simulink subsystem "EPOS4"  (R2021b)
settings: Solver=VariableStepAuto  StartTime=0.0  StopTime=10.0  RelTol=1e-3
undefined symbols (not defined in the file): DiscIntNeverNeededParam, Ts_Vel, x3001_5, x30A0_1, x30A0_2, x30A2_1, x30A2_2, x30A3_1, x30A3_2, x30A3_3, x30A3_4, x30A3_5, x520886_ICont, x607325_RotIner, x607325_RotOmgMax, x607325_Torq, x607325_TorqConst, x607325_VNom
libraries: fl_lib x4, nesl_utility x3, ee_lib x2, slpidlib x1
settings Model: Creator=khoi  LastModifiedBy=khoi
settings SolverCC: AlgebraicLoopSolver=TrustRegion
settings DebuggingCC: SFMachineParentedDataDiag=warning

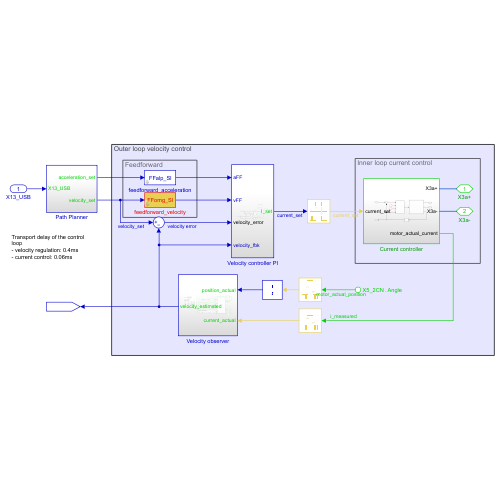
[thumbnail: Simulink's stored preview of the top-level diagram]
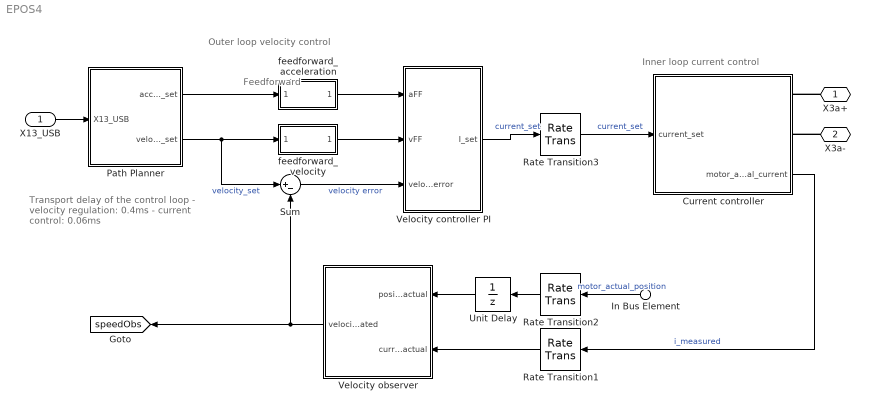
== system EPOS4 ==
  note: Outer loop velocity control
  note: Feedforward
  note: Inner loop current control
  note: Transport delay of the control loop
      | - velocity regulation: 0.4ms
      | - current control: 0.06ms
  X13_USB : Inport  OutDataTypeStr=double
  In Bus Element : Inport  Port=2  PortName=X5_2CN  Element=Angle
  Current controller : Subsystem
      settings: PortSchema="{\"entries\":[{\"content\":{\"sides\":[{\"content\":{\"connectorIds\":[\"In1\"]},\"type\":\"ConnectorPlacement.EquallySpacedRectSide\",\"uuid\":\"3e5704e1-1bc4-4e0c-b161-9fade073eb22\"},{\"content\":{\"connectorIds\":[\"RConn1\",\"RConn2\",\"Out1\"],\"side\":\"RIGHT\"},\"type\":\"ConnectorPlacement.EquallySpacedRectSide\",\"uuid\":\"52ff2dfd-ee16-417d-b7e8-bdd096001b9c\"},{\"content\":{\"connectorIds\":[],\"side\":\"TOP\"},\"type\":\"ConnectorPlacement.EquallySpacedRectSide\",\"uuid\":\"337a9011-df50-4122-8385-03af17ddf6d7\"}]},\"type\":\"ConnectorPlacement.EquallySpacedConnector\",\"uuid\":\"8d932baa-b47a-45b5-987d-77891fcdc649\"}],\"packageUris\":[\"http://schema.mathworks.com/mf0/Connector/R2020b\"],\"version\":\"1.0\"}"
  Path Planner : Subsystem
  Rate Transition1 : RateTransition  Deterministic=off  OutPortSampleTime=Ts_Vel
  Rate Transition2 : RateTransition  Deterministic=off  OutPortSampleTime=Ts_Vel
  Rate Transition3 : RateTransition  Deterministic=off  OutPortSampleTime=Ts_Curr
  Sum : Sum  Inputs=|+-
  Unit Delay : UnitDelay  SampleTime=Ts_Vel  HasFrameUpgradeWarning=on
  Velocity controller PI : Subsystem
  Velocity observer : Subsystem
  feedforward_acceleration : Subsystem  mask{Value=80}
      mask prompts: Value "Load inertia (g*cm^2)"
      mask TypeOptions Value: Constant1/Value
      mask DialogControl DescGroupVar Prompt: Feedforward acceleration
      mask Display: disp('FFalp_SI')
  feedforward_velocity : Subsystem  mask{Value=0}
      mask prompts: Value "Total friction proportional factor"
      mask DialogControl DescGroupVar Prompt: Feedforward velocity
      mask Display: disp('FFomg_SI')
  X3a+ : PMIOPort  Side=Left
  X3a- : PMIOPort  Port=2  Side=Left
  tag scope: speedObs=global
  wires:
  Path Planner/2(velocity_set) -> feedforward_velocity/1(X13_USB), Sum/1  "velocity_set"
  Path Planner/1(acceleration_set) -> feedforward_acceleration/1(X13_USB)
  feedforward_acceleration/1(Out1) -> Velocity controller PI/1(aFF)
  In Bus Element/1 -> Rate Transition2/1  "motor_actual_position"
  Current controller/1(motor_actual_current) -> Rate Transition1/1  "i_measured"
  feedforward_velocity/1(Out1) -> Velocity controller PI/2(vFF)
  Velocity controller PI/1(I_set) -> Rate Transition3/1  "current_set"
  Rate Transition3/1 -> Current controller/1(current_set)  "current_set"
  X13_USB/1 -> Path Planner/1(X13_USB)
  Unit Delay/1 -> Velocity observer/1(position_actual)
  Rate Transition2/1 -> Unit Delay/1
  Rate Transition1/1 -> Velocity observer/2(current_actual)
  Velocity observer/1(velocity_estimated) -> Sum/2, [speedObs]
  Sum/1 -> Velocity controller PI/3(velocity_error)  "velocity error"
  connections:
  X3a+/RConn1 -- Current controller/RConn1
  X3a-/RConn1 -- Current controller/RConn2

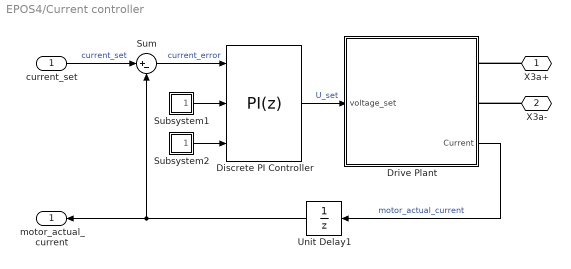
== system EPOS4/Current controller ==
  current_set : Inport  Unit=A
  Discrete PI Controller : slpidlib/PID Controller  Controller=PI  Form=Parallel  TimeDomain=Discrete-time  UseExternalTs=off  SampleTime=-1  IntegratorMethod=Forward Euler  FilterMethod=Forward Euler  ControllerParametersSource=external  P=1  I=1  D=0  UseFilter=on  N=100  TunerSelectOption=Transfer Function Based (PID Tuner App)  InitialConditionSource=internal  InitialConditionForIntegrator=0  InitialConditionForFilter=0  DifferentiatorICPrevScaledInput=0  ExternalReset=none  TrackingMode=off  Kt=0  LimitOutput=on  SatLimitsSource=internal  UpperSaturationLimit=x607325_VNom  LowerSaturationLimit=-x607325_VNom  LinearizeAsGain=off  AntiWindupMode=clamping  Kb=500  POutMin=[]  POutMax=[]  IOutMin=[]  IOutMax=[]  DOutMin=[]  DOutMax=[]  NOutMin=[]  NOutMax=[]  SumOutMin=[]  SumOutMax=[]  SaturationOutMin=[]  SaturationOutMax=[]  PParamMin=[]  PParamMax=[]  IParamMin=[]  IParamMax=[]  DParamMin=[]  DParamMax=[]  NParamMin=[]  NParamMax=[]  KbParamMin=[]  KbParamMax=[]  KtParamMin=[]  KtParamMax=[]  KbOutMin=[]  KbOutMax=[]  KtOutMin=[]  KtOutMax=[]  IntegratorOutMin=[]  IntegratorOutMax=[]  FilterOutMin=[]  FilterOutMax=[]  SumI1OutMin=[]  SumI1OutMax=[]  SumI2OutMin=[]  SumI2OutMax=[]  SumI3OutMin=[]  SumI3OutMax=[]  SumI4OutMin=[]  SumI4OutMax=[]  SumDOutMin=[]  SumDOutMax=[]  DifferentiatorOutMin=[]  DifferentiatorOutMax=[]  FilterDiffOutCoefMin=[]  FilterDiffOutCoefMax=[]  ReciprocalOutMin=[]  ReciprocalOutMax=[]  SumDenOutMin=[]  SumDenOutMax=[]  SumNumOutMin=[]  SumNumOutMax=[]  DivideOutMin=[]  DivideOutMax=[]  UdiffTsProdOutMin=[]  UdiffTsProdOutMax=[]  NTsProdOutMin=[]  NTsProdOutMax=[]  UintegralTsProdOutMin=[]  UintegralTsProdOutMax=[]  UngainTsProdOutMin=[]  UngainTsProdOutMax=[]  IntegratorContinuousStateAttributes=''  IntegratorStateMustResolveToSignalObject=off  IntegratorRTWStateStorageClass=Auto  FilterContinuousStateAttributes=''  FilterStateMustResolveToSignalObject=off  FilterRTWStateStorageClass=Auto  ParallelPVariant=ExternalParameters  IdealPVariant=Disabled  IVariant=ExternalParameters  DVariant=Disabled  IntegratorVariant=Discrete  SatVariant=Enabled  AWVariant=DiscClampingParallel  PCopyVariant=Disabled  TRVariant=Disabled  FdbkBlocksVariant=Forward  IdealPFdbkVariant=Disabled  SatFdbkVariant=Disabled  DerivativeFilterVariant=Disabled  NVariant=Disabled  NCopyVariant=Disabled_SignalSpec  FilterICVariant=Disabled  IntegratorICVariant=InternalICs  ExternalResetVariant=Disabled  TRSumVariant=Passthrough  SumFdbkVariant=Disabled  SumVariant=Sum_PI  TsampFilterVariant=InternalTs  TsampNgainVariant=Passthrough  TsampIntegralVariant=Passthrough  ExternalSaturationOutDataTypeStr=Inherit: Same as second input
  Drive Plant : Subsystem
      settings: PortSchema="{\"entries\":[{\"content\":{\"sides\":[{\"content\":{\"connectorIds\":[\"In1\"]},\"type\":\"ConnectorPlacement.EquallySpacedRectSide\",\"uuid\":\"2af1de9d-8962-474e-8952-77c9402ebadb\"},{\"content\":{\"connectorIds\":[\"RConn1\",\"RConn2\",\"Out1\"],\"side\":\"RIGHT\"},\"type\":\"ConnectorPlacement.EquallySpacedRectSide\",\"uuid\":\"e1a8f025-59c3-4187-9e1a-5d7de5437d6b\"},{\"content\":{\"connectorIds\":[],\"side\":\"TOP\"},\"type\":\"ConnectorPlacement.EquallySpacedRectSide\",\"uuid\":\"98ea0e18-1fc3-4a14-86ec-43c827e86c22\"}]},\"type\":\"ConnectorPlacement.EquallySpacedConnector\",\"uuid\":\"e2751f7d-b1df-4c60-a3ed-7b97aa6d6783\"}],\"packageUris\":[\"http://schema.mathworks.com/mf0/Connector/R2020b\"],\"version\":\"1.0\"}"
      mask Display: disp('Power\ndevice')
  Subsystem1 : Subsystem
  Subsystem2 : Subsystem
  Sum : Sum  Inputs=|+-
  Unit Delay1 : UnitDelay  SampleTime=0.06e-3  HasFrameUpgradeWarning=on
  X3a+ : PMIOPort  Side=Right
  X3a- : PMIOPort  Port=2  Side=Right
  motor_actual_current : Outport  Unit=A
  wires:
  current_set/1 -> Sum/1  "current_set"
  Subsystem2/1(Out1) -> Discrete PI Controller/3
  Subsystem1/1(Out1) -> Discrete PI Controller/2
  Unit Delay1/1 -> Sum/2, motor_actual_current/1
  Sum/1 -> Discrete PI Controller/1  "current_error"
  Discrete PI Controller/1 -> Drive Plant/1(voltage_set)  "U_set"
  Drive Plant/1(Current) -> Unit Delay1/1  "motor_actual_current"
  connections:
  X3a-/RConn1 -- Drive Plant/RConn2
  X3a+/RConn1 -- Drive Plant/RConn1

== system EPOS4/Path Planner ==
  X13_USB : Inport
  Demux : Demux  Outputs=3
  Terminator : Terminator
  acceleration_set : Outport  Unit=rad/s^2
  velocity_set : Outport  Port=2  Unit=rad/s
  wires:
  Demux/2 -> velocity_set/1
  X13_USB/1 -> Demux/1
  Demux/3 -> acceleration_set/1
  Demux/1 -> Terminator/1

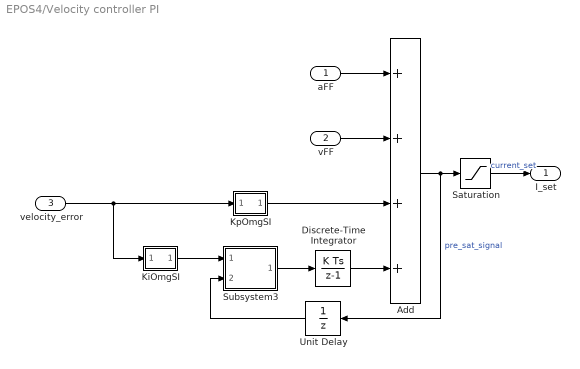
== system EPOS4/Velocity controller PI ==
  aFF : Inport
  vFF : Inport  Port=2
  velocity_error : Inport  Port=3  Unit=rad/s
  Add : Sum  Inputs=++++
  Discrete-Time Integrator : DiscreteIntegrator  SampleTime=-1  ICPrevOutput=DiscIntNeverNeededParam  ICPrevScaledInput=DiscIntNeverNeededParam
  KiOmgSI : Subsystem
  KpOmgSI : Subsystem
  Saturation : Saturate  UpperLimit=x520886_ICont  LowerLimit=-x520886_ICont
  Subsystem3 : Subsystem  mask{UpperValue=x520886_ICont, LowerValue=-x520886_ICont}
      mask prompts: UpperValue "Upper limit"; LowerValue "Lower limit"
      mask TypeOptions UpperValue: Dead Zone/UpperValue
      mask TypeOptions LowerValue: Dead Zone/LowerValue
      mask DialogControl DescGroupVar Prompt: Limit
      mask Display: disp('Anti-\nwindup')
  Unit Delay : UnitDelay  SampleTime=-1  HasFrameUpgradeWarning=on
  I_set : Outport  Unit=A
  wires:
  velocity_error/1 -> KpOmgSI/1(velocity_error), KiOmgSI/1(velocity_set)
  Add/1 -> Saturation/1, Unit Delay/1  "pre_sat_signal"
  KpOmgSI/1(Out1) -> Add/3
  vFF/1 -> Add/2
  KiOmgSI/1(Out1) -> Subsystem3/1(PreInt)
  aFF/1 -> Add/1
  Subsystem3/1(Out1) -> Discrete-Time Integrator/1
  Discrete-Time Integrator/1 -> Add/4
  Unit Delay/1 -> Subsystem3/2(PreSat)
  Saturation/1 -> I_set/1  "current_set"

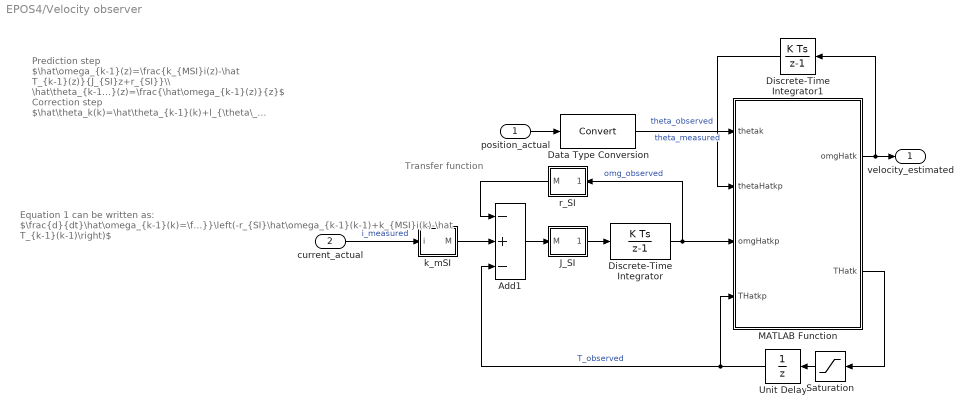
== system EPOS4/Velocity observer ==
  note: Prediction step
      | $\hat\omega_{k-1}(z)=\frac{k_{MSI}i(z)-\hat T_{k-1}(z)}{J_{SI}z+r_{SI}}\\ \hat\theta_{k-1}(z)=\frac{\hat\omega_{k-1}(z)}{z}$
      | Correction step
      | $\hat\theta_k(k)=\hat\theta_{k-1}(k)+l_{\theta\_ SI}\left[\theta(k)-\hat\theta_{k-1}(k)\right]\\ \hat\omega_k(k)=\hat\omega_{k-1}(k)+l_{\omega\_ SI}\left[\theta(k)-\hat\theta_{k}(k)\right]\\ \hat T_k(k)=\hat T_{k-1}(k)+l_{T\_ SI}\left[\theta(k)-\hat\theta_{k}(k)\right]\\$
  note: Equation 1 can be written as:
      | $\frac{d}{dt}\hat\omega_{k-1}(k)=\frac{1}{J_{SI}}\left(-r_{SI}\hat\omega_{k-1}(k-1)+k_{MSI}i(k)-\hat T_{k-1}(k-1)\right)$
  note: Transfer function
  position_actual : Inport  Unit=rad
  current_actual : Inport  Port=2  OutDataTypeStr=double
  Add1 : Sum  Inputs=-+-
  Data Type Conversion : DataTypeConversion
  Discrete-Time Integrator : DiscreteIntegrator  SampleTime=-1  LimitOutput=on  UpperSaturationLimit=x607325_RotOmgMax*pi/30  LowerSaturationLimit=-x607325_RotOmgMax*pi/30  ICPrevOutput=DiscIntNeverNeededParam  ICPrevScaledInput=DiscIntNeverNeededParam
  Discrete-Time Integrator1 : DiscreteIntegrator  SampleTime=-1  ICPrevOutput=DiscIntNeverNeededParam  ICPrevScaledInput=DiscIntNeverNeededParam
  J_SI : Subsystem
  MATLAB Function : MATLAB Function  TreatAsAtomicUnit=on  mask{lThetaSI=x30A3_1/1e3, lOmgSI=x30A3_2/1e3, lTSI=x30A3_3/1e6}
      mask prompts: lThetaSI "l_thetaSI"; lOmgSI "l_omgSI"; lTSI "l_TSI"
  Saturation : Saturate  UpperLimit=x607325_Torq/1e3  LowerLimit=-x607325_Torq/1e3
  Unit Delay : UnitDelay  SampleTime=-1  HasFrameUpgradeWarning=on
  k_mSI : Subsystem
  r_SI : Subsystem
  velocity_estimated : Outport  Unit=rad/s
  wires:
  Discrete-Time Integrator/1 -> MATLAB Function/3(omgHatkp), r_SI/1(dw_dt)  "omg_observed"
  Unit Delay/1 -> Add1/3, MATLAB Function/4(THatkp)  "T_observed"
  Saturation/1 -> Unit Delay/1
  J_SI/1(dw_dt) -> Discrete-Time Integrator/1
  r_SI/1(M) -> Add1/1
  k_mSI/1(M) -> Add1/2
  MATLAB Function/1(omgHatk) -> velocity_estimated/1, Discrete-Time Integrator1/1
  Add1/1 -> J_SI/1(M)
  current_actual/1 -> k_mSI/1(i)  "i_measured"
  Discrete-Time Integrator1/1 -> MATLAB Function/2(thetaHatkp)  "theta_observed"
  Data Type Conversion/1 -> MATLAB Function/1(thetak)  "theta_measured"
  position_actual/1 -> Data Type Conversion/1
  MATLAB Function/2(THatk) -> Saturation/1

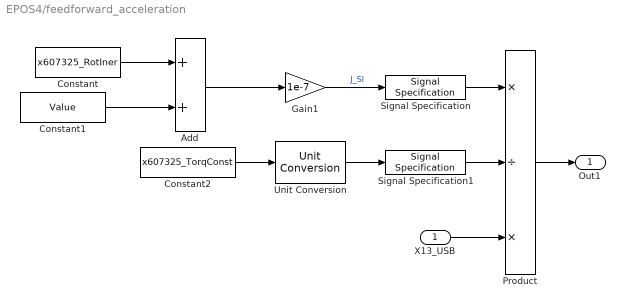
== system EPOS4/feedforward_acceleration ==
  X13_USB : Inport  Unit=rad/s^2
  Add : Sum
  Constant : Constant  Value=x607325_RotIner
  Constant1 : Constant  Value=Value
  Constant2 : Constant  Value=x607325_TorqConst
  Gain1 : Gain  Gain=1e-7
  Product : Product  Inputs=*/*
  Signal Specification : SignalSpecification  Unit=kg*m^2
  Signal Specification1 : SignalSpecification  Unit=N*m/A
  Unit Conversion : UnitConversion
  Out1 : Outport  Unit=A
  wires:
  Constant1/1 -> Add/2
  Constant2/1 -> Unit Conversion/1
  Gain1/1 -> Signal Specification/1  "J_SI"
  Product/1 -> Out1/1
  Add/1 -> Gain1/1
  Signal Specification1/1 -> Product/2
  X13_USB/1 -> Product/3
  Unit Conversion/1 -> Signal Specification1/1
  Constant/1 -> Add/1
  Signal Specification/1 -> Product/1

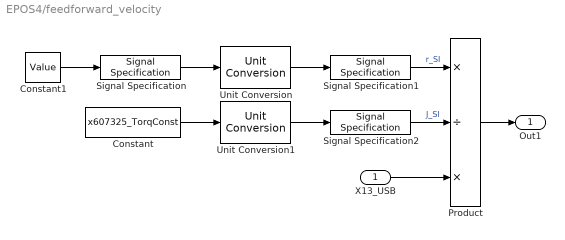
== system EPOS4/feedforward_velocity ==
  X13_USB : Inport  Unit=rad/s
  Constant : Constant  Value=x607325_TorqConst
  Constant1 : Constant  Value=Value
  Product : Product  Inputs=*/*
  Signal Specification : SignalSpecification  Unit=µN*m/(rpm)
  Signal Specification1 : SignalSpecification  Unit=N*m/(rad/s)
  Signal Specification2 : SignalSpecification  Unit=N*m/A
  Unit Conversion : UnitConversion
  Unit Conversion1 : UnitConversion
  Out1 : Outport  Unit=A
  wires:
  Unit Conversion1/1 -> Signal Specification2/1
  Signal Specification/1 -> Unit Conversion/1
  Unit Conversion/1 -> Signal Specification1/1
  Product/1 -> Out1/1
  Constant1/1 -> Signal Specification/1
  Constant/1 -> Unit Conversion1/1
  X13_USB/1 -> Product/3
  Signal Specification1/1 -> Product/1  "r_SI"
  Signal Specification2/1 -> Product/2  "J_SI"

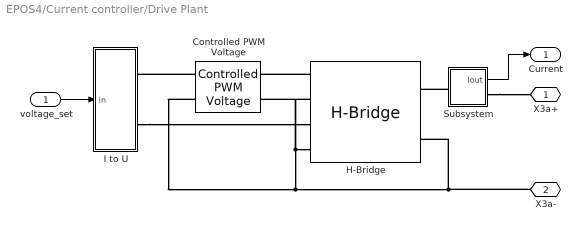
== system EPOS4/Current controller/Drive Plant ==
  voltage_set : Inport  Unit=V
  Controlled PWM Voltage : ee_lib/Integrated Circuits/Controlled PWM Voltage  F=20 kHz  TD=0 s  pulse_width_offset=0 s  pulse_min=0 s  pwm_or_av=2  event_type=1  sample_time=1e-6 s  Vmin=0 V  Vmax=x607325_VNom V  Vm=x607325_VNom V  u_min=0  u_max=1
  H-Bridge : ee_lib/Semiconductors & Converters/Converters/H-Bridge  supply_ports=ee.enum.supply_ports.hidesupply  pwm_or_av=ee.enum.pwm_or_av.averaged  regenerative_braking_mode=ee.enum.converters.regenerative_braking_mode.always_enabled  discontinuous=ee.enum.current_profile.continuous  freewheeling_mode=ee.enum.converters.freewheeling_mode.one_switch_one_diode  Rload=10 Ohm  Lload=1e-5 H  F=10 kHz  Venable=2.5 V  Vmax=x607325_VNom V  Vreverse=2.5 V  Vbrake=2.5 V  Vm=x607325_VNom V  Ron=0.1 Ohm  Don=0.1 Ohm  Goff=1e-6 S  Tmeas=298.15 K  Ron2=0.1 Ohm  Don2=0.05 Ohm  Tmeas2=398.15 K  thermal_mass=100 J/K  initial_temperature=298.15 K
  I to U : Subsystem
      mask Display: disp('V')
  Subsystem : Subsystem
  X3a+ : PMIOPort  Side=Right
  X3a- : PMIOPort  Port=2  Side=Right
  Current : Outport  Unit=A
  wires:
  Subsystem/1(Iout) -> Current/1
  voltage_set/1 -> I to U/1(in)
  connections:
  Subsystem/LConn1 -- H-Bridge/RConn1
  I to U/RConn2 -- H-Bridge/LConn3
  H-Bridge/LConn4 -- H-Bridge/LConn2 -- Controlled PWM Voltage/RConn2 -- X3a-/RConn1 -- H-Bridge/RConn2 -- Controlled PWM Voltage/LConn2
  H-Bridge/LConn1 -- Controlled PWM Voltage/RConn1
  Subsystem/RConn1 -- X3a+/RConn1
  Controlled PWM Voltage/LConn1 -- I to U/RConn1

== system EPOS4/Current controller/Subsystem1 ==
  Constant : Constant  Value=x30A0_1
  Signal Specification1 : SignalSpecification  Unit=V/A
  Unit Conversion : UnitConversion
  Out1 : Outport
  wires:
  Signal Specification1/1 -> Out1/1
  Unit Conversion/1 -> Signal Specification1/1
  Constant/1 -> Unit Conversion/1

== system EPOS4/Current controller/Subsystem2 ==
  Constant : Constant  Value=x30A0_2
  Signal Specification1 : SignalSpecification  Unit=V/(A*s)
  Unit Conversion : UnitConversion
  Out1 : Outport
  wires:
  Unit Conversion/1 -> Signal Specification1/1
  Signal Specification1/1 -> Out1/1
  Constant/1 -> Unit Conversion/1

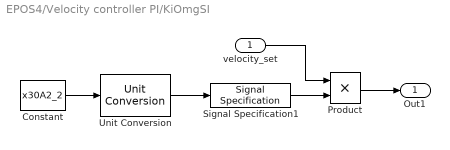
== system EPOS4/Velocity controller PI/KiOmgSI ==
  velocity_set : Inport  Unit=rad/s
  Constant : Constant  Value=x30A2_2
  Product : Product
  Signal Specification1 : SignalSpecification  Unit=A/rad
  Unit Conversion : UnitConversion
  Out1 : Outport  Unit=A/s
  wires:
  Constant/1 -> Unit Conversion/1
  Unit Conversion/1 -> Signal Specification1/1
  velocity_set/1 -> Product/1
  Product/1 -> Out1/1
  Signal Specification1/1 -> Product/2

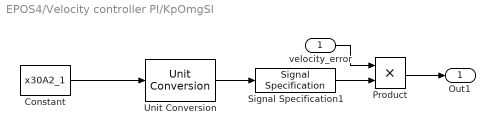
== system EPOS4/Velocity controller PI/KpOmgSI ==
  velocity_error : Inport  Unit=rad/s
  Constant : Constant  Value=x30A2_1
  Product : Product
  Signal Specification1 : SignalSpecification  Unit=A*s/rad
  Unit Conversion : UnitConversion
  Out1 : Outport  Unit=A
  wires:
  Product/1 -> Out1/1
  velocity_error/1 -> Product/1
  Signal Specification1/1 -> Product/2
  Constant/1 -> Unit Conversion/1
  Unit Conversion/1 -> Signal Specification1/1

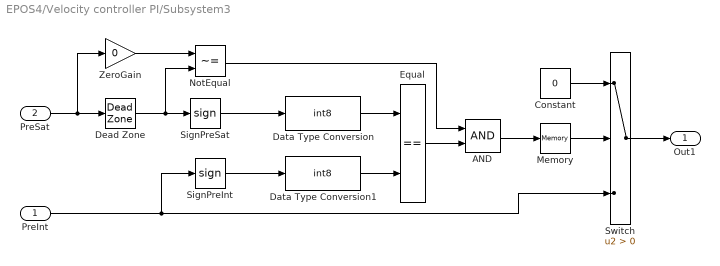
== system EPOS4/Velocity controller PI/Subsystem3 ==
  PreInt : Inport
  PreSat : Inport  Port=2
  AND : Logic  AllPortsSameDT=off  OutDataTypeStr=boolean
  Constant : Constant  Value=0
  Data Type Conversion : DataTypeConversion  OutDataTypeStr=int8  RndMeth=Simplest
  Data Type Conversion1 : DataTypeConversion  OutDataTypeStr=int8  RndMeth=Simplest
  Dead Zone : DeadZone  LowerValue=LowerValue  UpperValue=UpperValue  SaturateOnIntegerOverflow=on
  Equal : RelationalOperator  Operator===  OutDataTypeStr=boolean  RndMeth=Simplest
  Memory : Memory  DisableCoverage=on  InheritSampleTime=on
  NotEqual : RelationalOperator  DisableCoverage=on  Operator=~=  OutDataTypeStr=boolean
  SignPreInt : Signum
  SignPreSat : Signum
  Switch : Switch  Criteria=u2 > Threshold  InputSameDT=on
  ZeroGain : Gain  DisableCoverage=on  Gain=0  OutDataTypeStr=Inherit: Same as input  ParamDataTypeStr=Inherit: Same as input
  Out1 : Outport
  wires:
  Switch/1 -> Out1/1
  PreSat/1 -> ZeroGain/1, Dead Zone/1
  PreInt/1 -> SignPreInt/1, Switch/3
  Dead Zone/1 -> NotEqual/2, SignPreSat/1
  SignPreSat/1 -> Data Type Conversion/1
  AND/1 -> Memory/1
  Equal/1 -> AND/2
  Memory/1 -> Switch/2
  Constant/1 -> Switch/1
  SignPreInt/1 -> Data Type Conversion1/1
  Data Type Conversion1/1 -> Equal/2
  Data Type Conversion/1 -> Equal/1
  NotEqual/1 -> AND/1
  ZeroGain/1 -> NotEqual/1

== system EPOS4/Velocity observer/J_SI ==
  M : Inport  Unit=N*m*rad
  J_EPOS4 : Constant  Value=x30A3_5
  Product : Product  Inputs=*/
  Signal Specification1 : SignalSpecification  Unit=kg*m^2
  Unit Conversion : UnitConversion
  dw_dt : Outport  Unit=rad/s^2
  wires:
  M/1 -> Product/1
  Unit Conversion/1 -> Signal Specification1/1
  Signal Specification1/1 -> Product/2
  J_EPOS4/1 -> Unit Conversion/1
  Product/1 -> dw_dt/1

== system EPOS4/Velocity observer/k_mSI ==
  i : Inport  Unit=A
  Product : Product
  Signal Specification1 : SignalSpecification  Unit=N*m/A
  Unit Conversion : UnitConversion
  k_mEPOS4 : Constant  Value=x3001_5
  M : Outport  Unit=N*m
  wires:
  k_mEPOS4/1 -> Unit Conversion/1
  Product/1 -> M/1
  Unit Conversion/1 -> Signal Specification1/1
  i/1 -> Product/1
  Signal Specification1/1 -> Product/2

== system EPOS4/Velocity observer/r_SI ==
  dw_dt : Inport  Unit=rad/s
  Product : Product
  Signal Specification1 : SignalSpecification  Unit=N*m/(rad/s)
  Unit Conversion : UnitConversion
  r_EPOS4 : Constant  Value=x30A3_4
  M : Outport  Unit=N*m
  wires:
  dw_dt/1 -> Product/1
  Signal Specification1/1 -> Product/2
  Unit Conversion/1 -> Signal Specification1/1
  r_EPOS4/1 -> Unit Conversion/1
  Product/1 -> M/1

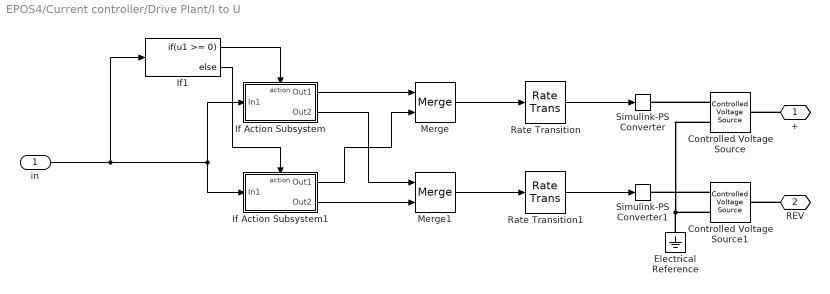
== system EPOS4/Current controller/Drive Plant/I to U ==
  in : Inport
  Controlled Voltage Source : fl_lib/Electrical/Electrical Sources/Controlled Voltage Source
  Controlled Voltage Source1 : fl_lib/Electrical/Electrical Sources/Controlled Voltage Source
  Electrical Reference : fl_lib/Electrical/Electrical Elements/Electrical Reference
  If Action Subsystem : Subsystem  TreatAsAtomicUnit=on
  If Action Subsystem1 : Subsystem  TreatAsAtomicUnit=on
  If1 : If  IfExpression=u1 >= 0
  Merge : Merge  InitialOutput=0
  Merge1 : Merge  InitialOutput=0
  Rate Transition : RateTransition
  Rate Transition1 : RateTransition
  Simulink-PS Converter : nesl_utility/Simulink-PS Converter  PhysicalDomain=network_engine_domain  SubClassName=ps_input  LeftPortType=input  RightPortType=output  PseudoPeriodic=off  Frequencies=[]  NoiseDistribution=none  NoiseParameters=[]  Unit=V  AffineConversion=off  FilteringAndDerivatives=provide  SimscapeFilterOrder=1  InputFilterTimeConstant=0.001  UdotUserProvided=0
  Simulink-PS Converter1 : nesl_utility/Simulink-PS Converter  PhysicalDomain=network_engine_domain  SubClassName=ps_input  LeftPortType=input  RightPortType=output  PseudoPeriodic=off  Frequencies=[]  NoiseDistribution=none  NoiseParameters=[]  Unit=V  AffineConversion=off  FilteringAndDerivatives=provide  SimscapeFilterOrder=1  InputFilterTimeConstant=0.001  UdotUserProvided=0
  + : PMIOPort  Side=Right
  REV : PMIOPort  Port=2  Side=Right
  wires:
  Rate Transition1/1 -> Simulink-PS Converter1/1
  Rate Transition/1 -> Simulink-PS Converter/1
  Merge1/1 -> Rate Transition1/1
  Merge/1 -> Rate Transition/1
  If Action Subsystem/1(Out1) -> Merge/1
  If1/2 -> If Action Subsystem1/Action
  If Action Subsystem1/2(Out2) -> Merge1/2
  If Action Subsystem/2(Out2) -> Merge1/1
  If Action Subsystem1/1(Out1) -> Merge/2
  If1/1 -> If Action Subsystem/Action
  in/1 -> If1/1, If Action Subsystem1/1(In1), If Action Subsystem/1(In1)
  connections:
  REV/RConn1 -- Controlled Voltage Source1/LConn1
  +/RConn1 -- Controlled Voltage Source/LConn1
  Controlled Voltage Source1/RConn1 -- Simulink-PS Converter1/RConn1
  Electrical Reference/LConn1 -- Controlled Voltage Source1/RConn2 -- Controlled Voltage Source/RConn2
  Controlled Voltage Source/RConn1 -- Simulink-PS Converter/RConn1

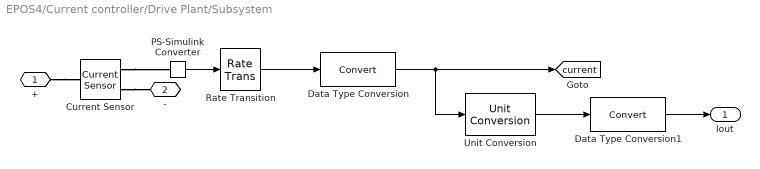
== system EPOS4/Current controller/Drive Plant/Subsystem ==
  Current Sensor : fl_lib/Electrical/Electrical Sensors/Current Sensor
  Data Type Conversion : DataTypeConversion
  Data Type Conversion1 : DataTypeConversion
  PS-Simulink Converter : nesl_utility/PS-Simulink Converter  PhysicalDomain=network_engine_domain  SubClassName=ps_output  LeftPortType=input  RightPortType=output  PseudoPeriodic=off  Frequencies=[]  Unit=inherit  AffineConversion=off
      settings: SourceProductBaseCode=PW,SS
  Rate Transition : RateTransition
  Unit Conversion : UnitConversion
  + : PMIOPort  Side=Left
  - : PMIOPort  Port=2  Side=Right
  Iout : Outport
  tag scope: current=global
  wires:
  Data Type Conversion1/1 -> Iout/1
  Rate Transition/1 -> Data Type Conversion/1
  Data Type Conversion/1 -> Unit Conversion/1, [current]
  Unit Conversion/1 -> Data Type Conversion1/1
  PS-Simulink Converter/1 -> Rate Transition/1
  connections:
  Current Sensor/RConn1 -- PS-Simulink Converter/LConn1
  +/RConn1 -- Current Sensor/LConn1
  Current Sensor/RConn2 -- -/RConn1

== system EPOS4/Current controller/Drive Plant/I to U/If Action Subsystem ==
  In1 : Inport
  Action Port : ActionPort
  Zero : Constant  Value=0  OutDataTypeStr=Inherit: Inherit via back propagation
  Out1 : Outport  Unit=V
  Out2 : Outport  Port=2  Unit=V
  wires:
  Zero/1 -> Out2/1
  In1/1 -> Out1/1

== system EPOS4/Current controller/Drive Plant/I to U/If Action Subsystem1 ==
  In1 : Inport
  Action Port : ActionPort
  Constant : Constant  Value=x607325_VNom
  Gain : Gain  Gain=-1  OutMin=-5  OutMax=5
  Out1 : Outport  Unit=V  SourceOfInitialOutputValue=Input signal
  Out2 : Outport  Port=2  Unit=V  SourceOfInitialOutputValue=Input signal  InitialOutput=0
  wires:
  Gain/1 -> Out1/1
  In1/1 -> Gain/1
  Constant/1 -> Out2/1

== matlab function EPOS4/Velocity observer/MATLAB Function ==
  data: omgHatk output; thetak input double; thetaHatkp input double; omgHatkp input double; THatkp input double; lTSI parameter; lOmgSI parameter; lThetaSI parameter; THatk output
function [omgHatk,THatk] = fCorrection(thetak, thetaHatkp, omgHatkp, THatkp,...
    lTSI, lOmgSI, lThetaSI)
    % Correction steps for prediction variables
    thetaHatk = thetaHatkp + lThetaSI*(thetak-thetaHatkp);
    omgHatk = omgHatkp + lOmgSI*(thetak-thetaHatk);
    THatk = THatkp + lTSI*(thetak-thetaHatk);
